simulink model "Static"  (R2015a)
settings: Solver=ode5  StartTime=0.0  StopTime=15  FixedStep=0.001  RelTol=1e-3
values from neighbouring files (symbols this model uses):
  a = 0.15    [Init.m]    (also in lyapu.m; plotKinematic.m = 0.13)
  a_e = (1 + err_a)*a    (= 0.15)    [Init.m]
  d = 0.05    [Init.m]    (also in plotKinematic.m = 0.1)
  K = 5    [Init.m]
  r = 0.1    [Init.m]    (also in plotKinematic.m)
  R = 2    [Init.m]
  r_e = (1 + err_r)*r    (= 0.1)    [Init.m]
  theta0 = pi    (= 3.14159265359)    [Init.m]
  wd = 0.5    [Init.m]
  x0 = 2.3    [Init.m]
  y0 = 0    [Init.m]
settings Model: Creator=tgvo  LastModifiedBy=tgvo
settings DataIOCC: LimitDataPoints=off

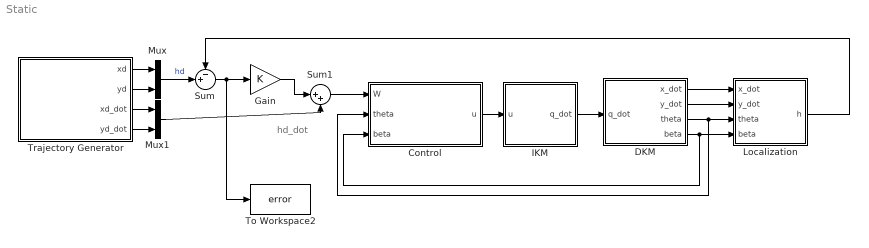
== system Static ==
  note: hd_dot
  Control : Subsystem  mask{a=a, d=d}
      mask prompts: a "Distance between steerable wheel and Om"; d "Distance between steearble wheel and tracking point"
  DKM : Subsystem  mask{a=a, r=r, theta0=theta0}
  Gain : Gain  Gain=K
  IKM : Subsystem  mask{a_e=a_e, r_e=r_e}
      mask prompts: a_e "Estimated distance b/w steerable wheel and Om"; r_e "Estimated wheel radius"
  Localization : Subsystem  mask{a=a, d=d, x0=x0, y0=y0}
      mask prompts: a "Distance b/w O_m and steerable wheel"; d "Distance b/w steerable wheel and tracking point"
  Mux : Mux  Inputs=2
  Mux1 : Mux  Inputs=2
  Sum : Sum  Inputs=-+|
  Sum1 : Sum  Inputs=|++
  To Workspace2 : ToWorkspace  VariableName=error  SampleTime=-1
  Trajectory Generator : Subsystem  mask{R=R, wd=wd}
      mask prompts: R "Radius of Circular Trajectory (R)"; wd "Desired Rotational Velocity (wd)"
  wires:
  Trajectory Generator/2(yd) -> Mux/2
  Trajectory Generator/1(xd) -> Mux/1
  Trajectory Generator/4(yd_dot) -> Mux1/2
  Trajectory Generator/3(xd_dot) -> Mux1/1
  Mux/1 -> Sum/2  "hd"
  Sum/1 -> To Workspace2/1, Gain/1
  Sum1/1 -> Control/1(W)
  Localization/1(h) -> Sum/1
  Gain/1 -> Sum1/1
  Mux1/1 -> Sum1/2
  IKM/1(q_dot) -> DKM/1(q_dot)
  Control/1(u) -> IKM/1(u)
  DKM/4(beta) -> Localization/4(beta), Control/3(beta)
  DKM/1(x_dot) -> Localization/1(x_dot)
  DKM/2(y_dot) -> Localization/2(y_dot)
  DKM/3(theta) -> Localization/3(theta), Control/2(theta)

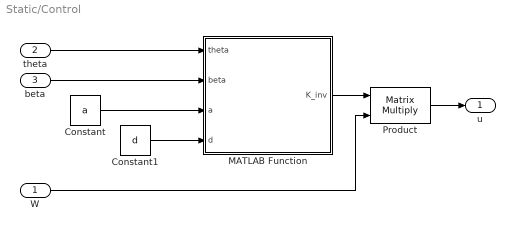
== system Static/Control ==
  W : Inport
  theta : Inport  Port=2
  beta : Inport  Port=3
  Constant : Constant  Value=a
  Constant1 : Constant  Value=d
  MATLAB Function : MATLAB Function  TreatAsAtomicUnit=on
  Product : Product  Multiplication=Matrix(*)
  u : Outport
  wires:
  beta/1 -> MATLAB Function/2(beta)
  W/1 -> Product/2
  Product/1 -> u/1
  theta/1 -> MATLAB Function/1(theta)
  Constant/1 -> MATLAB Function/3(a)
  Constant1/1 -> MATLAB Function/4(d)
  MATLAB Function/1(K_inv) -> Product/1

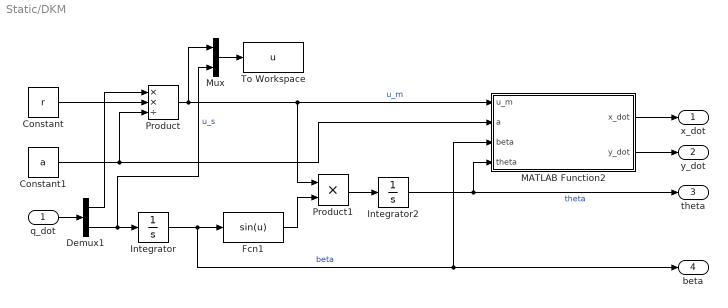
== system Static/DKM ==
  q_dot : Inport
  Constant : Constant  Value=r
  Constant1 : Constant  Value=a
  Demux1 : Demux  Outputs=2
  Fcn1 : Fcn  Expr=sin(u)
  Integrator : Integrator
  Integrator2 : Integrator  InitialCondition=theta0
  MATLAB Function2 : MATLAB Function  TreatAsAtomicUnit=on
  Mux : Mux  Inputs=2
  Product : Product  Inputs=**/
  Product1 : Product
  To Workspace : ToWorkspace  VariableName=u  SampleTime=-1
  x_dot : Outport
  y_dot : Outport  Port=2
  theta : Outport  Port=3
  beta : Outport  Port=4
  wires:
  Constant/1 -> Product/2
  Demux1/1 -> Product/1
  Integrator/1 -> MATLAB Function2/3(beta), beta/1, Fcn1/1  "beta"
  Fcn1/1 -> Product1/2
  Product/1 -> Product1/1, MATLAB Function2/1(u_m), Mux/1  "u_m"
  Product1/1 -> Integrator2/1
  q_dot/1 -> Demux1/1
  Demux1/2 -> Mux/2, Integrator/1  "u_s"
  Constant1/1 -> Product/3, MATLAB Function2/2(a)
  Integrator2/1 -> theta/1, MATLAB Function2/4(theta)  "theta"
  MATLAB Function2/2(y_dot) -> y_dot/1
  MATLAB Function2/1(x_dot) -> x_dot/1
  Mux/1 -> To Workspace/1

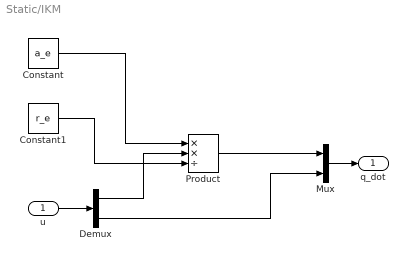
== system Static/IKM ==
  u : Inport
  Constant : Constant  Value=a_e
  Constant1 : Constant  Value=r_e
  Demux : Demux  Outputs=2
  Mux : Mux  Inputs=2
  Product : Product  Inputs=**/
  q_dot : Outport
  wires:
  u/1 -> Demux/1
  Constant/1 -> Product/1
  Demux/1 -> Product/2
  Constant1/1 -> Product/3
  Mux/1 -> q_dot/1
  Product/1 -> Mux/1
  Demux/2 -> Mux/2

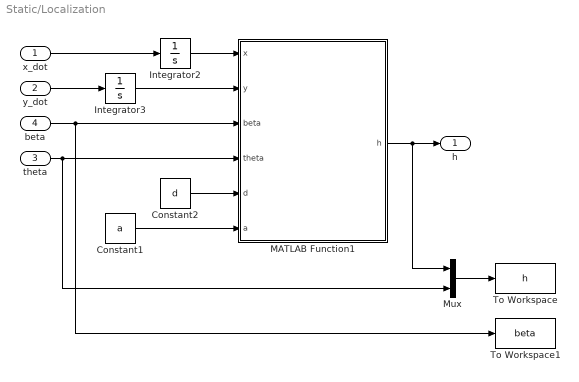
== system Static/Localization ==
  x_dot : Inport
  y_dot : Inport  Port=2
  theta : Inport  Port=3
  beta : Inport  Port=4
  Constant1 : Constant  Value=a
  Constant2 : Constant  Value=d
  Integrator2 : Integrator  InitialCondition=x0
  Integrator3 : Integrator  InitialCondition=y0
  MATLAB Function1 : MATLAB Function  TreatAsAtomicUnit=on
  Mux : Mux  Inputs=2
  To Workspace : ToWorkspace  VariableName=h  SampleTime=-1
  To Workspace1 : ToWorkspace  VariableName=beta  SampleTime=-1
  h : Outport
  wires:
  beta/1 -> To Workspace1/1, MATLAB Function1/3(beta)
  theta/1 -> Mux/2, MATLAB Function1/4(theta)
  x_dot/1 -> Integrator2/1
  y_dot/1 -> Integrator3/1
  Integrator2/1 -> MATLAB Function1/1(x)
  Integrator3/1 -> MATLAB Function1/2(y)
  Constant2/1 -> MATLAB Function1/5(d)
  MATLAB Function1/1(h) -> Mux/1, h/1
  Constant1/1 -> MATLAB Function1/6(a)
  Mux/1 -> To Workspace/1

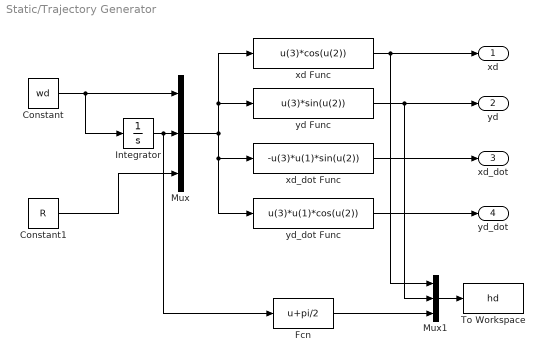
== system Static/Trajectory Generator ==
  Constant : Constant  Value=wd
  Constant1 : Constant  Value=R
  Fcn : Fcn  Expr=u+pi/2
  Integrator : Integrator
  Mux : Mux  Inputs=3
  Mux1 : Mux  Inputs=3
  To Workspace : ToWorkspace  VariableName=hd  SampleTime=-1
  xd Func : Fcn  Expr=u(3)*cos(u(2))
  xd_dot Func : Fcn  Expr=-u(3)*u(1)*sin(u(2))
  yd Func : Fcn  Expr=u(3)*sin(u(2))
  yd_dot Func : Fcn  Expr=u(3)*u(1)*cos(u(2))
  xd : Outport
  yd : Outport  Port=2
  xd_dot : Outport  Port=3
  yd_dot : Outport  Port=4
  wires:
  Constant1/1 -> Mux/3
  Mux/1 -> yd_dot Func/1, xd_dot Func/1, yd Func/1, xd Func/1
  yd_dot Func/1 -> yd_dot/1
  xd Func/1 -> Mux1/1, xd/1
  xd_dot Func/1 -> xd_dot/1
  yd Func/1 -> Mux1/2, yd/1
  Constant/1 -> Integrator/1, Mux/1
  Integrator/1 -> Fcn/1, Mux/2
  Mux1/1 -> To Workspace/1
  Fcn/1 -> Mux1/3

== matlab function Static/Control/MATLAB Function ==
  data: theta input; K_inv output; beta input; a input; d input
function K_inv = Find_K_inv(theta,beta,a,d)
%#codegen

K = [a*cos(beta+theta)-d*sin(beta+theta)*sin(beta), -d*sin(beta+theta);...
     a*sin(beta+theta)+d*cos(beta+theta)*sin(beta), d*cos(beta+theta)];
 
 K_inv = inv(K);

== matlab function Static/Localization/MATLAB Function1 ==
  data: x input; y input; beta input; theta input; d input; a input; h output
function h = Find_h(x,y,beta,theta,d,a)
%#codegen
z1 = x + a*cos(theta) + d*cos(theta+beta);
z2 = y + a*sin(theta) + d*sin(theta+beta);
h = [z1;z2];

== matlab function Static/DKM/MATLAB Function2 ==
  data: u_m input; x_dot output; a input; beta input; theta input; y_dot output
function [x_dot,y_dot] = Find_xy_dot(u_m,a,beta,theta)

x_dot = a*cos(beta)*cos(theta)*u_m;
y_dot = a*cos(beta)*sin(theta)*u_m;
